simulink model "Mass_Spring_Dumper_System"  (R2025b)
settings: Solver=VariableStepAuto  StartTime=0.0  StopTime=100  MaxStep=0.01  RelTol=1e-3
InitFcn:
  | b = 0.1;
  | k = 20;
  | F = 1;
  | M = 1;
CloseFcn:
  | data = [out.simout.Time, out.simout.Data];
  | filename = fullfile('Simulations', 'Intro_To_Simulink', 'test.xlsx');
  | writematrix(data, filename);  % Creates real XLSX spreadsheet
settings Model: Creator=night  LastModifiedBy=night

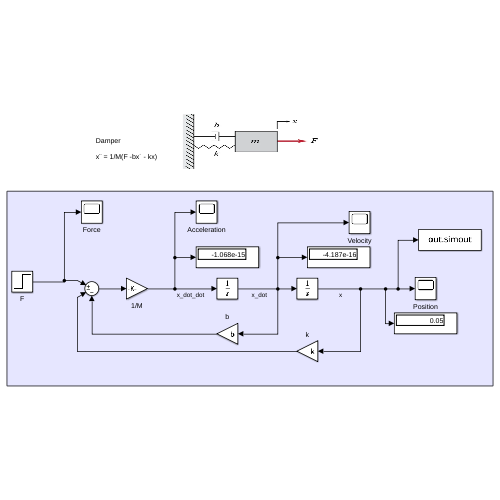
[thumbnail: Simulink's stored preview of the top-level diagram]
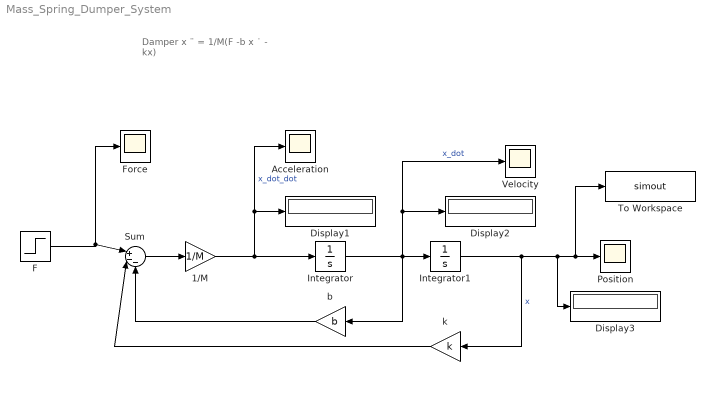
== system Mass_Spring_Dumper_System ==
  note: Damper
      |
      | x ¨ = 1/M(F -b x ˙ - kx)
  1/M : Gain  Gain=1/M
  Acceleration : Scope
      settings: ActiveDisplayYMinimum=-0.2557767844056249  ActiveDisplayYMaximum=1.1395307538228472  DataLoggingVariableName=ScopeData2
  Display1 : Display
  Display2 : Display
  Display3 : Display
  F : Step  InitFcn=|  Time=0  After=F  SampleTime=0
      | b = 0.1;
      | k = 20;
      | F = 1;
      | M = 1;
  Force : Scope
      settings: ActiveDisplayYMinimum=-1  ActiveDisplayYMaximum=1  DataLoggingVariableName=ScopeData3
  Integrator : Integrator
  Integrator1 : Integrator
  Position : Scope
      settings: ActiveDisplayYMinimum=-0.012283444059675585  ActiveDisplayYMaximum=0.1105509965370803
  Sum : Sum  Inputs=|+--
  To Workspace : ToWorkspace  VariableName=simout  SaveFormat=Timeseries  SampleTime=-1
  Velocity : Scope
      settings: ActiveDisplayYMinimum=-0.00952765756915498  ActiveDisplayYMaximum=0.085748918122394838
  b : Gain  Gain=b
  k : Gain  Gain=k
  wires:
  1/M/1 -> Acceleration/1, Display1/1, Integrator/1  "x_dot_dot"
  Integrator/1 -> b/1, Velocity/1, Display2/1, Integrator1/1  "x_dot"
  Integrator1/1 -> k/1, Display3/1, To Workspace/1, Position/1  "x"
  F/1 -> Force/1, Sum/1
  b/1 -> Sum/3
  k/1 -> Sum/2
  Sum/1 -> 1/M/1
